simulink model "Vent_Ctrl_01"  (R2022a)
settings: Solver=VariableStepAuto  StartTime=0.0  StopTime=10.0  RelTol=1e-3
libraries: simulink x2
settings Model: Creator=smith  LastModifiedBy=smith

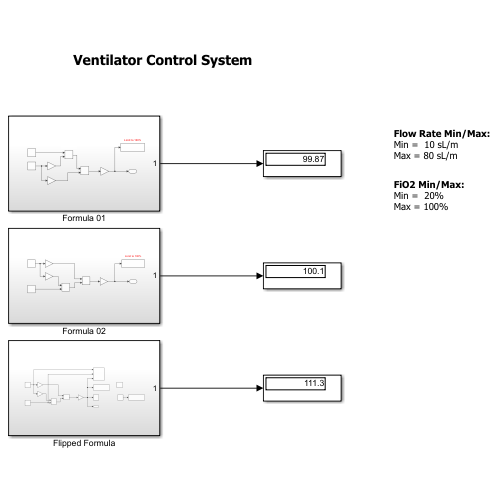
[thumbnail: Simulink's stored preview of the top-level diagram]
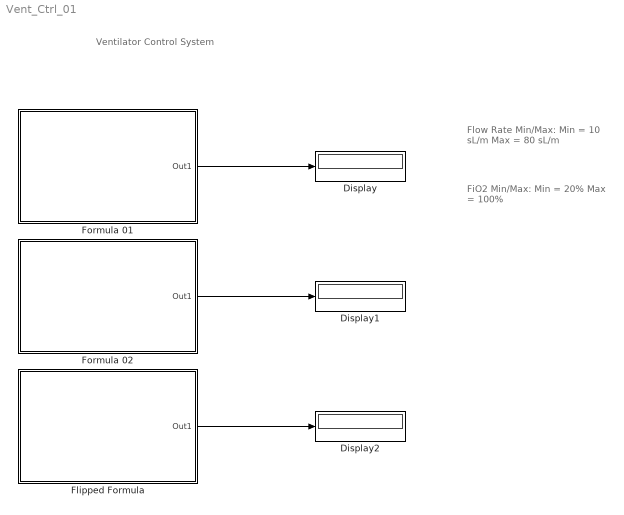
== system Vent_Ctrl_01 ==
  note: Flow Rate Min/Max:
      | Min = 10 sL/m
      | Max = 80 sL/m
  note: Ventilator Control System
  note: FiO2 Min/Max:
      | Min = 20%
      | Max = 100%
  Display : Display
  Display1 : Display
  Display2 : Display
  Flipped Formula : Subsystem
  Formula 01 : Subsystem
  Formula 02 : Subsystem
  wires:
  Formula 01/1(Out1) -> Display/1
  Formula 02/1(Out1) -> Display1/1
  Flipped Formula/1(Out1) -> Display2/1

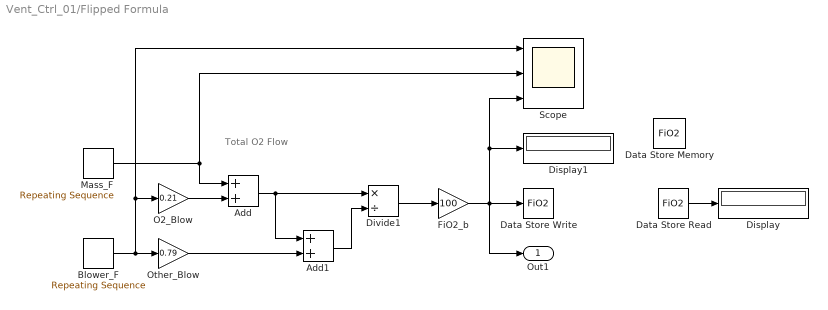
== system Vent_Ctrl_01/Flipped Formula ==
  note: Total
      | O2 Flow
  Add : Sum
  Add1 : Sum
  Blower_F : simulink/Sources/Repeating Sequence  rep_seq_t=[0 1 1.1 2 2.1 3 3.1 4 4.1]  rep_seq_y=[20 20 50 50 35 35 45 45 20]
  Data Store Memory : DataStoreMemory  DataStoreName=FiO2  WriteAfterWriteMsg=warning  ShowAdditionalParam=off
  Data Store Read : DataStoreRead  DataStoreName=FiO2  IndexOptions=Index vector (dialog)  Indices=1  OutputSizes=1
  Data Store Write : DataStoreWrite  DataStoreName=FiO2  IndexOptions=Index vector (dialog)  Indices=1  OutputSizes=1
  Display : Display
  Display1 : Display
  Divide1 : Product  Inputs=*/
  FiO2_b : Gain  Gain=100
  Mass_F : simulink/Sources/Repeating Sequence  rep_seq_t=[0 1 1.1 2 2.1 3 3.1 4 4.1]  rep_seq_y=[10 10 25 25 50 50 40 40 10]
  O2_Blow : Gain  Gain=0.21
  Other_Blow : Gain  Gain=0.79
  Scope : Scope  NumInputPorts=3
  Out1 : Outport
  wires:
  Data Store Read/1 -> Display/1
  FiO2_b/1 -> Scope/3, Display1/1, Data Store Write/1, Out1/1
  Divide1/1 -> FiO2_b/1
  Blower_F/1 -> Scope/1, O2_Blow/1, Other_Blow/1
  Mass_F/1 -> Scope/2, Add/1
  Add/1 -> Divide1/1, Add1/1
  Other_Blow/1 -> Add1/2
  O2_Blow/1 -> Add/2
  Add1/1 -> Divide1/2

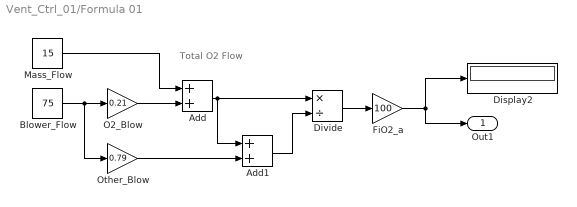
== system Vent_Ctrl_01/Formula 01 ==
  note: Total
      | O2 Flow
  Add : Sum
  Add1 : Sum
  Blower_Flow : Constant  Value=75
  Display2 : Display
  Divide : Product  Inputs=*/
  FiO2_a : Gain  Gain=100
  Mass_Flow : Constant  Value=15
  O2_Blow : Gain  Gain=0.21
  Other_Blow : Gain  Gain=0.79
  Out1 : Outport
  wires:
  Divide/1 -> FiO2_a/1
  FiO2_a/1 -> Out1/1, Display2/1
  O2_Blow/1 -> Add/2
  Mass_Flow/1 -> Add/1
  Blower_Flow/1 -> Other_Blow/1, O2_Blow/1
  Add/1 -> Add1/1, Divide/1
  Add1/1 -> Divide/2
  Other_Blow/1 -> Add1/2

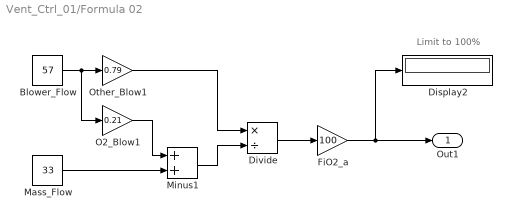
== system Vent_Ctrl_01/Formula 02 ==
  note: Limit to 100%
  Blower_Flow : Constant  Value=57
  Display2 : Display
  Divide : Product  Inputs=*/
  FiO2_a : Gain  Gain=100
  Mass_Flow : Constant  Value=33
  Minus1 : Sum
  O2_Blow1 : Gain  Gain=0.21
  Other_Blow1 : Gain  Gain=0.79
  Out1 : Outport
  wires:
  Minus1/1 -> Divide/2
  FiO2_a/1 -> Out1/1, Display2/1
  Divide/1 -> FiO2_a/1
  Blower_Flow/1 -> O2_Blow1/1, Other_Blow1/1
  O2_Blow1/1 -> Minus1/1
  Other_Blow1/1 -> Divide/1
  Mass_Flow/1 -> Minus1/2
